simulink model "simple_streaming_txrx"  (Simulink 6.6)
settings: Solver=ode45  StartTime=0.0  StopTime=inf  RelTol=1e-3
InitFcn:
  | simple_streaming_init
StartFcn:
  | simple_streaming_init
undefined symbols (not defined in the file): dmf, gcbh, get, modConstellation_qam16, modConstellation_qam64, modConstellation_qpsk, rcosfir, symbolRomLen, txLSFR_initValues, txLSFR_polynomials, viqAvgLen, xlBlockLoadCallback, xlGetSimulinkPeriod
libraries: xbsIndex_r4 x506, commchan3 x2, commsink2 x1
(part 3 of 5)

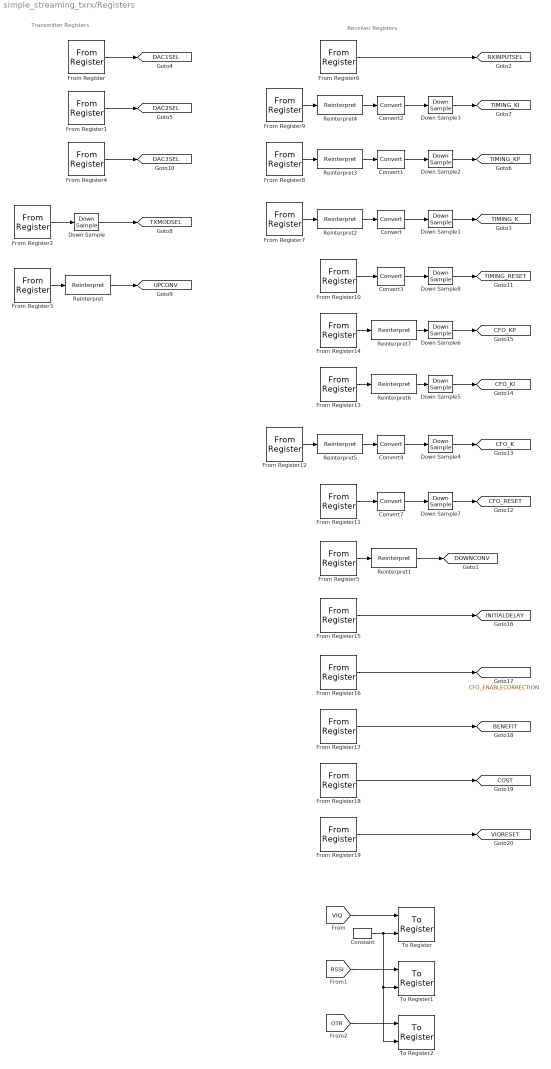
== system simple_streaming_txrx/Registers ==
  note: Transmitter Registers
  note: Receiver Registers
  Constant : xbsIndex_r4/Constant  arith_type=Boolean  const=1  n_bits=16  bin_pt=14  explicit_period=off  period=1  equ=P=C  opselect=C  inp2=PCIN>>17  opr=+  inp1=P  carry=CIN  dbl_ovrd=off  block_type=constant
      settings: block_version=10.1.2
  Convert : xbsIndex_r4/Convert  arith_type=Unsigned  n_bits=17  bin_pt=14  quantization=Truncate  overflow=Wrap  latency=0  dbl_ovrd=off  pipeline=off  block_type=convert
      settings: xl_area=[0 0 0 0 0 0 0]  block_version=10.1
  Convert1 : xbsIndex_r4/Convert  arith_type=Unsigned  n_bits=34  bin_pt=34  quantization=Truncate  overflow=Wrap  latency=0  dbl_ovrd=off  pipeline=off  block_type=convert
      settings: xl_area=[0 0 0 0 0 0 0]  block_version=10.1
  Convert2 : xbsIndex_r4/Convert  arith_type=Unsigned  n_bits=34  bin_pt=34  quantization=Truncate  overflow=Wrap  latency=0  dbl_ovrd=off  pipeline=off  block_type=convert
      settings: xl_area=[0 0 0 0 0 0 0]  block_version=10.1
  Convert3 : xbsIndex_r4/Convert  arith_type=Boolean  n_bits=17  bin_pt=14  quantization=Truncate  overflow=Wrap  latency=0  dbl_ovrd=off  pipeline=off  block_type=convert
      settings: xl_area=[0 0 0 0 0 0 0]  block_version=10.1
  Convert4 : xbsIndex_r4/Convert  arith_type=Unsigned  n_bits=17  bin_pt=10  quantization=Truncate  overflow=Wrap  latency=0  dbl_ovrd=off  pipeline=off  block_type=convert
      settings: xl_area=[0 0 0 0 0 0 0]  block_version=10.1
  Convert7 : xbsIndex_r4/Convert  arith_type=Boolean  n_bits=17  bin_pt=14  quantization=Truncate  overflow=Wrap  latency=0  dbl_ovrd=off  pipeline=off  block_type=convert
      settings: xl_area=[0 0 0 0 0 0 0]  block_version=10.1
  Down Sample{,1..8} (9 alike) : xbsIndex_r4/Down Sample  sample_ratio=8  sample_phase="Last Value of Frame  (most efficient)"  en=off  latency=1  dbl_ovrd=off  block_type=dsamp
      Down Sample settings: xl_area=[1 2 0 0 0 0 0]  block_version=10.1
      Down Sample1 settings: xl_area=[9 17 0 0 0 0 0]  block_version=10.1
      Down Sample2 settings: xl_area=[17 34 0 0 0 0 0]  block_version=10.1
      Down Sample3 settings: xl_area=[17 34 0 0 0 0 0]  block_version=10.1
      Down Sample4 settings: xl_area=[9 17 0 0 0 0 0]  block_version=10.1
      Down Sample5 settings: xl_area=[16 32 0 0 0 0 0]  block_version=10.1
      Down Sample6 settings: xl_area=[16 32 0 0 0 0 0]  block_version=10.1
      Down Sample7 settings: xl_area=[1 1 0 0 0 0 0]  block_version=10.1
      Down Sample8 settings: xl_area=[1 1 0 0 0 0 0]  block_version=10.1
  From Register : xbsIndex_r4/From Register  shared_memory_name='dac1Sel'  init=dac1Sel  period=1/8  ownership=Locally owned and initialized  arith_type=Unsigned  n_bits=2  bin_pt=0  dbl_ovrd=off  block_type=fromreg
      settings: AttributesFormatString=<< %<shared_memory_name> >>  infoedit="Register block that reads data to a shared memory register.  Delay of one sample period."  block_version=10.1
  From Register1 : xbsIndex_r4/From Register  shared_memory_name='dac2Sel'  init=dac2Sel  period=1/8  ownership=Locally owned and initialized  arith_type=Unsigned  n_bits=2  bin_pt=0  dbl_ovrd=off  block_type=fromreg
      settings: AttributesFormatString=<< %<shared_memory_name> >>  infoedit="Register block that reads data to a shared memory register.  Delay of one sample period."  block_version=10.1
  From Register10 : xbsIndex_r4/From Register  shared_memory_name='timingReset'  init=timingReset  period=1/8  ownership=Locally owned and initialized  arith_type=Unsigned  n_bits=1  bin_pt=0  dbl_ovrd=off  block_type=fromreg
      settings: AttributesFormatString=<< %<shared_memory_name> >>  infoedit="Register block that reads data to a shared memory register.  Delay of one sample period."  block_version=10.1
  From Register11 : xbsIndex_r4/From Register  shared_memory_name='cfoReset'  init=cfoReset  period=1/8  ownership=Locally owned and initialized  arith_type=Unsigned  n_bits=1  bin_pt=0  dbl_ovrd=off  block_type=fromreg
      settings: AttributesFormatString=<< %<shared_memory_name> >>  infoedit="Register block that reads data to a shared memory register.  Delay of one sample period."  block_version=10.1
  From Register12 : xbsIndex_r4/From Register  shared_memory_name='cfoK'  init=cfoK  period=1/8  ownership=Locally owned and initialized  arith_type=Unsigned  n_bits=32  bin_pt=0  dbl_ovrd=off  block_type=fromreg
      settings: AttributesFormatString=<< %<shared_memory_name> >>  infoedit="Register block that reads data to a shared memory register.  Delay of one sample period."  block_version=10.1
  From Register13 : xbsIndex_r4/From Register  shared_memory_name='cfoKI'  init=cfoKI  period=1/8  ownership=Locally owned and initialized  arith_type=Unsigned  n_bits=32  bin_pt=0  dbl_ovrd=off  block_type=fromreg
      settings: AttributesFormatString=<< %<shared_memory_name> >>  infoedit="Register block that reads data to a shared memory register.  Delay of one sample period."  block_version=10.1
  From Register14 : xbsIndex_r4/From Register  shared_memory_name='cfoKP'  init=cfoKP  period=1/8  ownership=Locally owned and initialized  arith_type=Unsigned  n_bits=32  bin_pt=0  dbl_ovrd=off  block_type=fromreg
      settings: AttributesFormatString=<< %<shared_memory_name> >>  infoedit="Register block that reads data to a shared memory register.  Delay of one sample period."  block_version=10.1
  From Register15 : xbsIndex_r4/From Register  shared_memory_name='initialDelay'  init=initialDelay  period=1/8  ownership=Locally owned and initialized  arith_type=Unsigned  n_bits=2  bin_pt=0  dbl_ovrd=off  block_type=fromreg
      settings: AttributesFormatString=<< %<shared_memory_name> >>  infoedit="Register block that reads data to a shared memory register.  Delay of one sample period."  block_version=10.1
  From Register16 : xbsIndex_r4/From Register  shared_memory_name='cfoEnable'  init=cfoEnable  period=1/8  ownership=Locally owned and initialized  arith_type=Unsigned  n_bits=1  bin_pt=0  dbl_ovrd=off  block_type=fromreg
      settings: AttributesFormatString=<< %<shared_memory_name> >>  infoedit="Register block that reads data to a shared memory register.  Delay of one sample period."  block_version=10.1
  From Register17 : xbsIndex_r4/From Register  shared_memory_name='otrBenefit'  init=benefit  period=1/8  ownership=Locally owned and initialized  arith_type=Unsigned  n_bits=32  bin_pt=0  dbl_ovrd=off  block_type=fromreg
      settings: AttributesFormatString=<< %<shared_memory_name> >>  infoedit="Register block that reads data to a shared memory register.  Delay of one sample period."  block_version=10.1
  From Register18 : xbsIndex_r4/From Register  shared_memory_name='otrCost'  init=cost  period=1/8  ownership=Locally owned and initialized  arith_type=Unsigned  n_bits=32  bin_pt=0  dbl_ovrd=off  block_type=fromreg
      settings: AttributesFormatString=<< %<shared_memory_name> >>  infoedit="Register block that reads data to a shared memory register.  Delay of one sample period."  block_version=10.1
  From Register19 : xbsIndex_r4/From Register  shared_memory_name='viqReset'  init=0  period=1/8  ownership=Locally owned and initialized  arith_type=Unsigned  n_bits=1  bin_pt=0  dbl_ovrd=off  block_type=fromreg
      settings: AttributesFormatString=<< %<shared_memory_name> >>  infoedit="Register block that reads data to a shared memory register.  Delay of one sample period."  block_version=10.1
  From Register2 : xbsIndex_r4/From Register  shared_memory_name='txModSel'  init=txModSel  period=1/8  ownership=Locally owned and initialized  arith_type=Unsigned  n_bits=2  bin_pt=0  dbl_ovrd=off  block_type=fromreg
      settings: AttributesFormatString=<< %<shared_memory_name> >>  infoedit="Register block that reads data to a shared memory register.  Delay of one sample period."  block_version=10.1
  From Register3 : xbsIndex_r4/From Register  shared_memory_name='upConv'  init=upConv  period=1/8  ownership=Locally owned and initialized  arith_type=Unsigned  n_bits=32  bin_pt=0  dbl_ovrd=off  block_type=fromreg
      settings: AttributesFormatString=<< %<shared_memory_name> >>  infoedit="Register block that reads data to a shared memory register.  Delay of one sample period."  block_version=10.1
  From Register4 : xbsIndex_r4/From Register  shared_memory_name='dac3Sel'  init=dac3Sel  period=1/8  ownership=Locally owned and initialized  arith_type=Unsigned  n_bits=1  bin_pt=0  dbl_ovrd=off  block_type=fromreg
      settings: AttributesFormatString=<< %<shared_memory_name> >>  infoedit="Register block that reads data to a shared memory register.  Delay of one sample period."  block_version=10.1
  From Register5 : xbsIndex_r4/From Register  shared_memory_name='downConv'  init=downConv  period=1/8  ownership=Locally owned and initialized  arith_type=Unsigned  n_bits=32  bin_pt=0  dbl_ovrd=off  block_type=fromreg
      settings: AttributesFormatString=<< %<shared_memory_name> >>  infoedit="Register block that reads data to a shared memory register.  Delay of one sample period."  block_version=10.1
  From Register6 : xbsIndex_r4/From Register  shared_memory_name='rxInputSel'  init=rxInputSel  period=1/8  ownership=Locally owned and initialized  arith_type=Unsigned  n_bits=2  bin_pt=0  dbl_ovrd=off  block_type=fromreg
      settings: AttributesFormatString=<< %<shared_memory_name> >>  infoedit="Register block that reads data to a shared memory register.  Delay of one sample period."  block_version=10.1
  From Register7 : xbsIndex_r4/From Register  shared_memory_name='timingK'  init=timingK  period=1/8  ownership=Locally owned and initialized  arith_type=Unsigned  n_bits=32  bin_pt=0  dbl_ovrd=off  block_type=fromreg
      settings: AttributesFormatString=<< %<shared_memory_name> >>  infoedit="Register block that reads data to a shared memory register.  Delay of one sample period."  block_version=10.1
  From Register8 : xbsIndex_r4/From Register  shared_memory_name='timingKP'  init=timingKP  period=1/8  ownership=Locally owned and initialized  arith_type=Unsigned  n_bits=32  bin_pt=0  dbl_ovrd=off  block_type=fromreg
      settings: AttributesFormatString=<< %<shared_memory_name> >>  infoedit="Register block that reads data to a shared memory register.  Delay of one sample period."  block_version=10.1
  From Register9 : xbsIndex_r4/From Register  shared_memory_name='timingKI'  init=timingKI  period=1/8  ownership=Locally owned and initialized  arith_type=Unsigned  n_bits=32  bin_pt=0  dbl_ovrd=off  block_type=fromreg
      settings: AttributesFormatString=<< %<shared_memory_name> >>  infoedit="Register block that reads data to a shared memory register.  Delay of one sample period."  block_version=10.1
  Reinterpret{,1,3..4,6..7} (6 alike) : xbsIndex_r4/Reinterpret  force_arith_type=on  arith_type=Unsigned  force_bin_pt=on  bin_pt=32  block_type=reinterpret
      settings: infoedit="Changes signal type without altering the binary representation.   You can changed the signal between signed and unsigned, and relocate the binary point.<P><P>Hardware notes: In hardware this block costs nothing.<P><P>Example:  Suppose the input is 6 bits wide, signed, with 2 fractional bits, and the output is forced to unsigned with 0 fractional bits.  Then an input of -2.0 (1110.00 in binary 2's complement) becomes an output of 56 (111000 in binary)."  block_version=10.1
  Reinterpret2 : xbsIndex_r4/Reinterpret  force_arith_type=on  arith_type=Unsigned  force_bin_pt=on  bin_pt=29  block_type=reinterpret
      settings: infoedit="Changes signal type without altering the binary representation.   You can changed the signal between signed and unsigned, and relocate the binary point.<P><P>Hardware notes: In hardware this block costs nothing.<P><P>Example:  Suppose the input is 6 bits wide, signed, with 2 fractional bits, and the output is forced to unsigned with 0 fractional bits.  Then an input of -2.0 (1110.00 in binary 2's complement) becomes an output of 56 (111000 in binary)."  block_version=10.1
  Reinterpret5 : xbsIndex_r4/Reinterpret  force_arith_type=on  arith_type=Unsigned  force_bin_pt=on  bin_pt=25  block_type=reinterpret
      settings: infoedit="Changes signal type without altering the binary representation.   You can changed the signal between signed and unsigned, and relocate the binary point.<P><P>Hardware notes: In hardware this block costs nothing.<P><P>Example:  Suppose the input is 6 bits wide, signed, with 2 fractional bits, and the output is forced to unsigned with 0 fractional bits.  Then an input of -2.0 (1110.00 in binary 2's complement) becomes an output of 56 (111000 in binary)."  block_version=10.1
  To Register : xbsIndex_r4/To Register  shared_memory_name='viq'  init=0  ownership=Locally owned and initialized  explicit_data_type=on  arith_type=Unsigned  n_bits=32  bin_pt=0  dbl_ovrd=off  block_type=toreg
      settings: AttributesFormatString=<< %<shared_memory_name> >>  infoedit="Register block that writes data to a shared memory register.  Delay of one sample period."  block_version=10.1.2
  To Register1 : xbsIndex_r4/To Register  shared_memory_name='rssi'  init=0  ownership=Locally owned and initialized  explicit_data_type=on  arith_type=Unsigned  n_bits=32  bin_pt=0  dbl_ovrd=off  block_type=toreg
      settings: AttributesFormatString=<< %<shared_memory_name> >>  infoedit="Register block that writes data to a shared memory register.  Delay of one sample period."  block_version=10.1.2
  To Register2 : xbsIndex_r4/To Register  shared_memory_name='otr'  init=0  ownership=Locally owned and initialized  explicit_data_type=on  arith_type=Unsigned  n_bits=32  bin_pt=0  dbl_ovrd=off  block_type=toreg
      settings: AttributesFormatString=<< %<shared_memory_name> >>  infoedit="Register block that writes data to a shared memory register.  Delay of one sample period."  block_version=10.1.2
  tag scope: BENEFIT=global, CFO_ENABLECORRECTION=global, CFO_K=global, CFO_KI=global, CFO_KP=global, CFO_RESET=global, COST=global, DAC1SEL=global, DAC2SEL=global, DAC3SEL=global, DOWNCONV=global, INITIALDELAY=global, RXINPUTSEL=global, TIMING_K=global, TIMING_KI=global, TIMING_KP=global, TIMING_RESET=global, TXMODSEL=global, UPCONV=global, VIQRESET=global
  wires:
  From Register/1 -> [DAC1SEL]
  From Register1/1 -> [DAC2SEL]
  From Register2/1 -> Down Sample/1
  Down Sample/1 -> [TXMODSEL]
  From Register3/1 -> Reinterpret/1
  Reinterpret/1 -> [UPCONV]
  From Register4/1 -> [DAC3SEL]
  From Register5/1 -> Reinterpret1/1
  Reinterpret1/1 -> [DOWNCONV]
  From Register6/1 -> [RXINPUTSEL]
  From Register7/1 -> Reinterpret2/1
  Reinterpret2/1 -> Convert/1
  Convert/1 -> Down Sample1/1
  From Register8/1 -> Reinterpret3/1
  Reinterpret3/1 -> Convert1/1
  Convert1/1 -> Down Sample2/1
  From Register9/1 -> Reinterpret4/1
  Reinterpret4/1 -> Convert2/1
  Convert2/1 -> Down Sample3/1
  From Register10/1 -> Convert3/1
  Convert3/1 -> Down Sample8/1
  Down Sample1/1 -> [TIMING_K]
  Down Sample2/1 -> [TIMING_KP]
  Down Sample3/1 -> [TIMING_KI]
  From Register12/1 -> Reinterpret5/1
  Reinterpret5/1 -> Convert4/1
  Convert4/1 -> Down Sample4/1
  From Register13/1 -> Reinterpret6/1
  Reinterpret6/1 -> Down Sample5/1
  From Register14/1 -> Reinterpret7/1
  Reinterpret7/1 -> Down Sample6/1
  From Register11/1 -> Convert7/1
  Convert7/1 -> Down Sample7/1
  Down Sample4/1 -> [CFO_K]
  Down Sample5/1 -> [CFO_KI]
  Down Sample6/1 -> [CFO_KP]
  Down Sample7/1 -> [CFO_RESET]
  Down Sample8/1 -> [TIMING_RESET]
  From Register15/1 -> [INITIALDELAY]
  From Register16/1 -> [CFO_ENABLECORRECTION]
  From Register17/1 -> [BENEFIT]
  From Register18/1 -> [COST]
  [VIQ] -> To Register/1
  [RSSI] -> To Register1/1
  [OTR] -> To Register2/1
  Constant/1 -> To Register1/2, To Register2/2, To Register/2
  From Register19/1 -> [VIQRESET]

== system simple_streaming_txrx/Transmitter ==
  Interpolate : Subsystem
  Random Symbols : Subsystem
  Register : xbsIndex_r4/Register  init=0  rst=off  en=off  dbl_ovrd=off  block_type=register
      settings: xl_area=[8 16 0 0 0 0 0]  block_version=10.1
  Register1 : xbsIndex_r4/Register  init=0  rst=off  en=off  dbl_ovrd=off  block_type=register
      settings: xl_area=[8 16 0 0 0 0 0]  block_version=10.1
  TX_I : xbsIndex_r4/Gateway Out  hdl_port=on  timing_constraint=None  locs_specified=off  LOCs={}  block_type=gatewayout
      settings: infoedit="Gateway out block.  Converts Xilinx fixed point inputs into ouputs of type Simulink integer, double, or fixed point.<P><P>Hardware notes:  In hardware these blocks become top level output ports or are discarded, depending on how they are configured."  xl_area=[0 0 0 0 16 0 0]  block_version=10.1
  TX_Q : xbsIndex_r4/Gateway Out  hdl_port=on  timing_constraint=None  locs_specified=off  LOCs={}  block_type=gatewayout
      settings: infoedit="Gateway out block.  Converts Xilinx fixed point inputs into ouputs of type Simulink integer, double, or fixed point.<P><P>Hardware notes:  In hardware these blocks become top level output ports or are discarded, depending on how they are configured."  xl_area=[0 0 0 0 16 0 0]  block_version=10.1
  Upconverter : Subsystem
  Upconverted : Outport
  IF I : Outport  Port=2
  IF Q : Outport  Port=3
  tag scope: Symbols_Filt_I=global, Symbols_Filt_Q=global, Symbols_Tx_I=global, Symbols_Tx_Q=global, Upconverted=global
  wires:
  Random Symbols/1(I) -> [Symbols_Tx_I], Interpolate/1(I)
  Random Symbols/2(Q) -> [Symbols_Tx_Q], Interpolate/2(Q)
  Interpolate/1(" I") -> [Symbols_Filt_I], Upconverter/1(I)
  Interpolate/2(" Q") -> [Symbols_Filt_Q], Upconverter/2(Q)
  Upconverter/1(" Mixed") -> [Upconverted], Upconverted/1
  Upconverter/2(" I") -> Register/1
  Upconverter/3(" Q") -> Register1/1
  TX_I/1 -> IF I/1
  TX_Q/1 -> IF Q/1
  Register/1 -> TX_I/1
  Register1/1 -> TX_Q/1

== system simple_streaming_txrx/Receiver/AGC Hook ==
  I : Inport
  Q : Inport  Port=2
  Coarse : Subsystem
  Fine : Subsystem
  IO : Outport
  OO : Outport  Port=2
  wires:
  I/1 -> IO/1, Fine/1(I)
  Q/1 -> OO/1, Fine/2(Q)

== system simple_streaming_txrx/Receiver/Carrier Recovery ==
  I : Inport
  Q : Inport  Port=2
  2nd Order Filter : Subsystem
  Convert : xbsIndex_r4/Convert  arith_type=Boolean  n_bits=16  bin_pt=14  quantization=Truncate  overflow=Wrap  latency=0  dbl_ovrd=off  pipeline=off  block_type=convert
      settings: xl_area=[0 0 0 0 0 0 0]  block_version=10.1
  Inverter : xbsIndex_r4/Inverter  en=off  latency=0  dbl_ovrd=off  block_type=inv
      settings: xl_area=[0 0 0 0 0 0 0]  block_version=10.1
  Mult2 : xbsIndex_r4/Mult  precision=User Defined  arith_type="Signed  (2's comp)"  n_bits=32  bin_pt=31  quantization=Truncate  overflow=Flag as error  en=off  latency=3  dbl_ovrd=off  use_behavioral_HDL=off  use_embedded=on  opt=Speed  optimum_pipeline=off  pipeline=on  use_rpm=on  placement_style=Rectangular shape  block_type=mult
      settings: infoedit=Hardware notes: To use the internal pipeline stage of the dedicated multiplier you must select 'Pipeline for maximum performance'.  xl_area=[59 104 0 100 0 3 0]  block_version=10.1
  Phase Error Detector : Subsystem
  Register : xbsIndex_r4/Register  init=0  rst=on  en=off  dbl_ovrd=off  block_type=register
      settings: xl_area=[16 32 0 0 0 0 0]  block_version=10.1
  Up Sample : xbsIndex_r4/Up Sample  sample_ratio=8  copy_samples=on  dbl_ovrd=off  block_type=usamp
      settings: infoedit="Up samples input data.  Inserted values  can be zeros or copies of the most recent input sample.<P><P>Hardware notes: No hardware is needed if inserted values are copies of the input sample; otherwise, a mux and single bit flip-flop are used."  xl_area=[0 0 0 0 0 0 0]  block_version=10.1
  " phase inc" : Outport
  tag scope: CFOINC=global, PHASEERROR=global
  wires:
  Phase Error Detector/1(Err) -> 2nd Order Filter/1(Phase Error), [PHASEERROR]
  [CFO_RESET] -> 2nd Order Filter/2(Reset)
  Up Sample/1 -> Register/1
  2nd Order Filter/1(Phase Inc) -> Mult2/1
  I/1 -> Phase Error Detector/1(I)
  Q/1 -> Phase Error Detector/2(Q)
  [CFO_K] -> Mult2/2
  Mult2/1 -> Up Sample/1, [CFOINC]
  Register/1 -> " phase inc"/1
  [CFO_ENABLECORRECTION] -> Inverter/1
  Inverter/1 -> Convert/1
  Convert/1 -> Register/2

== system simple_streaming_txrx/Receiver/Decimate & Filter ==
  I : Inport
  Q : Inport  Port=2
  Convert1 : xbsIndex_r4/Convert  arith_type="Signed  (2's comp)"  n_bits=16  bin_pt=15  quantization=Truncate  overflow=Wrap  latency=0  dbl_ovrd=off  pipeline=off  block_type=convert
      settings: xl_area=[0 0 0 0 0 0 0]  block_version=10.1
  Convert2 : xbsIndex_r4/Convert  arith_type="Signed  (2's comp)"  n_bits=16  bin_pt=15  quantization=Truncate  overflow=Wrap  latency=0  dbl_ovrd=off  pipeline=off  block_type=convert
      settings: xl_area=[0 0 0 0 0 0 0]  block_version=10.1
  Convert3 : xbsIndex_r4/Convert  arith_type="Signed  (2's comp)"  n_bits=16  bin_pt=15  quantization=Truncate  overflow=Wrap  latency=0  dbl_ovrd=off  pipeline=off  block_type=convert
      settings: xl_area=[0 0 0 0 0 0 0]  block_version=10.1
  I MF1 : Subsystem  mask{h_in=rcosfir(.3, 4, 8, 1,'sqrt'), polyphaseBranches=8, data_samplePeriod=1/8, coeff_prec=14, coeff_bp=13, multLatency=1, mult_prec=18, mult_bp=17, add_prec=16, add_bp=14}
      mask prompts: h_in "Filter Coefficients"; polyphaseBranches "Interpolation Rate"; data_samplePeriod "Input Sample Period"; coeff_prec "Coefficients - Num Bits"; coeff_bp "Coefficients - Binary Point"; multLatency "Multiplier Latency"; mult_prec "Multiplier - Num Bits"; mult_bp "Multiplier - Binary Point"; add_prec "Final Adder - Num Bits"; add_bp "Final Adder - Binary Point"
      mask help:
      | This block implements a decimating polyphase FIR filter. In this version,
      | the decimation rate must be 8, and the filter must be of length 64.
      mask init:
      | h = reshape(reshape(h_in(1:64),8,8)',1,64);
      | subFilterLength = 8;
  I MF2 : Subsystem  mask{h_in=rcosfir(.3, 4, 8, 1,'sqrt'), polyphaseBranches=8, data_samplePeriod=1/8, coeff_prec=14, coeff_bp=13, multLatency=1, mult_prec=18, mult_bp=17, add_prec=16, add_bp=14}
      mask prompts: h_in "Filter Coefficients"; polyphaseBranches "Interpolation Rate"; data_samplePeriod "Input Sample Period"; coeff_prec "Coefficients - Num Bits"; coeff_bp "Coefficients - Binary Point"; multLatency "Multiplier Latency"; mult_prec "Multiplier - Num Bits"; mult_bp "Multiplier - Binary Point"; add_prec "Final Adder - Num Bits"; add_bp "Final Adder - Binary Point"
      mask help:
      | This block implements a decimating polyphase FIR filter. In this version,
      | the decimation rate must be 8, and the filter must be of length 64.
      mask init:
      | h = reshape(reshape(h_in(1:64),8,8)',1,64);
      | subFilterLength = 8;
  Scale : xbsIndex_r4/Scale  scale_factor=1  dbl_ovrd=off  block_type=scale
      settings: infoedit=Scales input by a power of two by adjusting the binary point position.<P><P>Hardware notes: In hardware this block costs nothing.  block_version=10.1
  Scale1 : xbsIndex_r4/Scale  scale_factor=0  dbl_ovrd=off  block_type=scale
      settings: infoedit=Scales input by a power of two by adjusting the binary point position.<P><P>Hardware notes: In hardware this block costs nothing.  block_version=10.1
  Scale2 : xbsIndex_r4/Scale  scale_factor=1  dbl_ovrd=off  block_type=scale
      settings: infoedit=Scales input by a power of two by adjusting the binary point position.<P><P>Hardware notes: In hardware this block costs nothing.  block_version=10.1
  Scope : Scope  NumInputPorts=6
      settings: YMin=-0.75~-0.75~-1~-1.5~-1.5~-1  YMax=0.75~0.75~0.75~1.5~1.5~0.75  SaveName=ScopeData4
  dMF : Subsystem  mask{h_in=dmf*2, polyphaseBranches=8, data_samplePeriod=1/8, coeff_prec=14, coeff_bp=13, multLatency=1, mult_prec=18, mult_bp=17, add_prec=16, add_bp=14}
      mask prompts: h_in "Filter Coefficients"; polyphaseBranches "Interpolation Rate"; data_samplePeriod "Input Sample Period"; coeff_prec "Coefficients - Num Bits"; coeff_bp "Coefficients - Binary Point"; multLatency "Multiplier Latency"; mult_prec "Multiplier - Num Bits"; mult_bp "Multiplier - Binary Point"; add_prec "Final Adder - Num Bits"; add_bp "Final Adder - Binary Point"
      mask help:
      | This block implements a decimating polyphase FIR filter. In this version,
      | the decimation rate must be 8, and the filter must be of length 64.
      mask init:
      | h = reshape(reshape(h_in(1:64),8,8)',1,64);
      | subFilterLength = 8;
  " I" : Outport
  " Q" : Outport  Port=2
  " dI" : Outport  Port=3
  wires:
  I/1 -> I MF1/1(X), dMF/1(X)
  I MF1/1(Y) -> Scale/1, Scope/1
  Q/1 -> I MF2/1(X)
  Scale/1 -> Convert3/1, Scope/4
  Scale2/1 -> Convert1/1, Scope/5
  Convert3/1 -> " I"/1
  Convert1/1 -> " Q"/1
  I MF2/1(Y) -> Scale2/1, Scope/2
  dMF/1(Y) -> Scale1/1, Scope/3
  Scale1/1 -> Convert2/1, Scope/6
  Convert2/1 -> " dI"/1

== system simple_streaming_txrx/Receiver/Downconverter ==
  Mixed : Inport
  SEL : Inport  Port=2
  I : Inport  Port=3
  Q : Inport  Port=4
  Phase Inc : Inport  Port=5
  AddSub : xbsIndex_r4/AddSub  mode=Addition  use_carryin=off  use_carryout=off  en=off  latency=0  precision=User Defined  arith_type=Unsigned  n_bits=32  bin_pt=32  quantization=Truncate  overflow=Wrap  dbl_ovrd=off  use_behavioral_HDL=on  pipelined=off  use_rpm=on  block_type=addsub
      settings: xl_area=[16 0 0 31 0 0 0]  block_version=10.1
  ComplexMult : Subsystem
  Inverter1 : xbsIndex_r4/Inverter  en=off  latency=0  dbl_ovrd=off  block_type=inv
      settings: xl_area=[0 0 0 0 0 0 0]  block_version=10.1
  Mux1 : xbsIndex_r4/Mux  inputs=3  en=off  latency=1  precision=Full  arith_type="Signed  (2's comp)"  n_bits=8  bin_pt=2  quantization=Truncate  overflow=Wrap  dbl_ovrd=off  block_type=mux
      settings: xl_area=[18 18 0 36 0 0 0]  block_version=10.1
  Mux2 : xbsIndex_r4/Mux  inputs=3  en=off  latency=1  precision=Full  arith_type="Signed  (2's comp)"  n_bits=8  bin_pt=2  quantization=Truncate  overflow=Wrap  dbl_ovrd=off  block_type=mux
      settings: xl_area=[18 18 0 36 0 0 0]  block_version=10.1
  i1i1 : xbsIndex_r4/Mult  precision=User Defined  arith_type="Signed  (2's comp)"  n_bits=18  bin_pt=17  quantization=Truncate  overflow=Flag as error  en=off  latency=1  dbl_ovrd=off  use_behavioral_HDL=off  use_embedded=on  opt=Speed  optimum_pipeline=off  pipeline=on  use_rpm=on  placement_style=Rectangular shape  block_type=mult
      settings: infoedit=Hardware notes: To use the internal pipeline stage of the dedicated multiplier you must select 'Pipeline for maximum performance'.  xl_area=[9 -11 0 18 0 1 0]  block_version=10.1
  i1i2 : xbsIndex_r4/Mult  precision=User Defined  arith_type="Signed  (2's comp)"  n_bits=18  bin_pt=17  quantization=Truncate  overflow=Flag as error  en=off  latency=1  dbl_ovrd=off  use_behavioral_HDL=off  use_embedded=on  opt=Speed  optimum_pipeline=off  pipeline=on  use_rpm=on  placement_style=Rectangular shape  block_type=mult
      settings: infoedit=Hardware notes: To use the internal pipeline stage of the dedicated multiplier you must select 'Pipeline for maximum performance'.  xl_area=[9 -11 0 18 0 1 0]  block_version=10.1
  myDDS : Subsystem
  " I" : Outport
  " Q" : Outport  Port=2
  tag scope: dCarrier_I=global
  wires:
  Mixed/1 -> i1i2/1, i1i1/1
  AddSub/1 -> myDDS/1(phase inc)
  Phase Inc/1 -> AddSub/2
  [DOWNCONV] -> AddSub/1
  myDDS/1(sin) -> Inverter1/1
  myDDS/2(cos) -> i1i2/2, [dCarrier_I], ComplexMult/1(A I)
  Mux1/1 -> " I"/1
  Mux2/1 -> " Q"/1
  SEL/1 -> Mux1/1, Mux2/1
  i1i2/1 -> Mux1/3, Mux1/2
  i1i1/1 -> Mux2/3, Mux2/2
  I/1 -> ComplexMult/3(B I)
  Q/1 -> ComplexMult/4(B Q)
  ComplexMult/1(I) -> Mux1/4
  ComplexMult/2(Q) -> Mux2/4
  Inverter1/1 -> i1i1/2, ComplexMult/2(A Q)

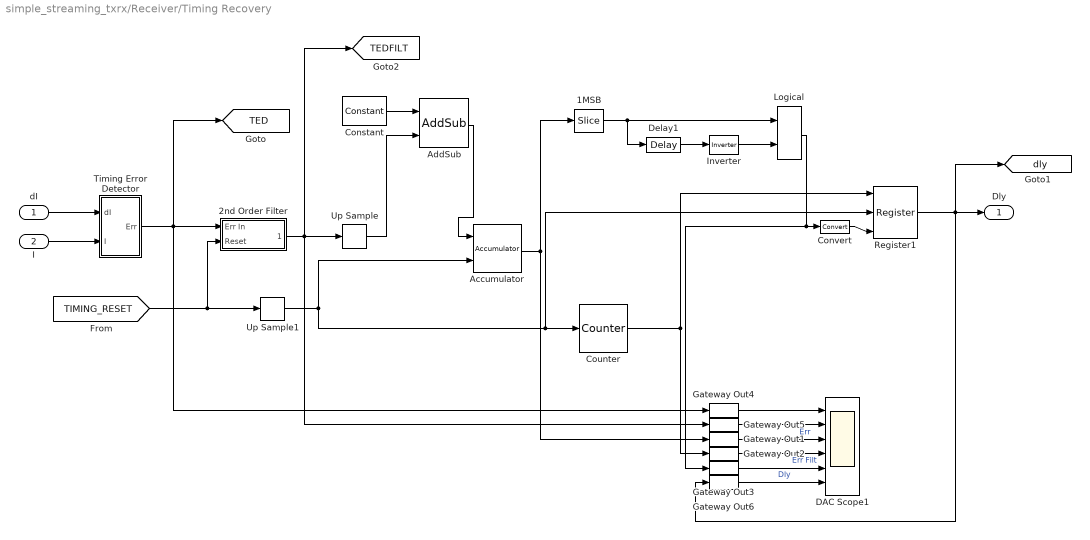
== system simple_streaming_txrx/Receiver/Timing Recovery ==
  dI : Inport
  I : Inport  Port=2
  1MSB : xbsIndex_r4/Slice  nbits=1  boolean_output=off  mode=Upper Bit Location + Width  bit1=0  base1=MSB of Input  bit0=0  base0=LSB of Input  dbl_ovrd=off  block_type=slice
      settings: infoedit="Extracts a given range of bits from each input sample and presents it at the output.  The output type is ordinarily unsigned with binary point at zero, but can be Boolean when the slice is one bit wide.<P><P>Hardware notes: In hardware this block costs nothing."  block_version=10.1
  2nd Order Filter : Subsystem
  Accumulator : xbsIndex_r4/Accumulator  operation=Add  n_bits=32  overflow=Wrap  scale=1  rst=on  hasbypass=off  en=off  dbl_ovrd=off  use_behavioral_HDL=on  block_type=accum
      settings: infoedit="Adder or subtractor-based accumulator.   Output type and binary point position match the input.<P><P>Hardware notes: When \"Reinitialize with input 'b' on reset\" is selected, the accumulator is forced to run at the system rate even if the input 'b' is running at a slower rate."  xl_area=[16 32 0 32 0 0 0]  block_version=10.1
  AddSub : xbsIndex_r4/AddSub  mode=Subtraction  use_carryin=off  use_carryout=off  en=off  latency=0  precision=User Defined  arith_type="Signed  (2's comp)"  n_bits=32  bin_pt=31  quantization=Truncate  overflow=Wrap  dbl_ovrd=off  use_behavioral_HDL=on  pipelined=off  use_rpm=on  block_type=addsub
      settings: xl_area=[2 0 0 4 0 0 0]  block_version=10.1
  Constant : xbsIndex_r4/Constant  arith_type=Unsigned  const=1/4  n_bits=4  bin_pt=3  explicit_period=on  period=1/8  equ=P=C  opselect=C  inp2=PCIN>>17  opr=+  inp1=P  carry=CIN  dbl_ovrd=off  block_type=constant
      settings: block_version=10.1
  Convert : xbsIndex_r4/Convert  arith_type=Boolean  n_bits=8  bin_pt=6  quantization=Truncate  overflow=Wrap  latency=0  dbl_ovrd=off  pipeline=off  block_type=convert
      settings: xl_area=[0 0 0 0 0 0 0]  block_version=10.1
  Counter : xbsIndex_r4/Counter  cnt_type=Free Running  cnt_to=Inf  operation=Up  start_count=0  cnt_by_val=1  arith_type=Unsigned  n_bits=3  bin_pt=0  load_pin=off  rst=on  en=off  explicit_period=off  period=1/8  dbl_ovrd=off  use_behavioral_HDL=off  use_rpm=on  block_type=counter
      settings: xl_area=[3 3 0 3 0 0 0]  block_version=10.1
  DAC Scope1 : Scope  NumInputPorts=6
      settings: YMin=-0.4~-0.0075~-1~0~0~-1  YMax=0.4~0.0075~1~7~1~1  SaveName=ScopeData3
  Delay1 : xbsIndex_r4/Delay  en=off  latency=1  dbl_ovrd=off  reg_retiming=off  block_type=delay
      settings: xl_area=[1 1 0 0 0 0 0]  block_version=10.1
  Gateway Out{1..6} (6 alike) : xbsIndex_r4/Gateway Out  hdl_port=off  timing_constraint=None  locs_specified=off  LOCs={}  block_type=gatewayout
      settings: infoedit="Gateway out block.  Converts Xilinx fixed point inputs into ouputs of type Simulink integer, double, or fixed point.<P><P>Hardware notes:  In hardware these blocks become top level output ports or are discarded, depending on how they are configured."  xl_area=[0 0 0 0 0 0 0]  block_version=10.1
  Inverter : xbsIndex_r4/Inverter  en=off  latency=0  dbl_ovrd=off  block_type=inv
      settings: xl_area=[0 0 0 0 0 0 0]  block_version=10.1
  Logical : xbsIndex_r4/Logical  logical_function=AND  inputs=2  en=off  latency=0  precision=Full  arith_type=Unsigned  n_bits=8  bin_pt=2  align_bp=on  dbl_ovrd=off  block_type=logical
      settings: xl_area=[1 0 0 1 0 0 0]  block_version=10.1
  Register1 : xbsIndex_r4/Register  init=0  rst=on  en=on  dbl_ovrd=off  block_type=register
      settings: xl_area=[2 3 0 0 0 0 0]  block_version=10.1
  Timing Error Detector : Subsystem
  Up Sample : xbsIndex_r4/Up Sample  sample_ratio=8  copy_samples=on  dbl_ovrd=off  block_type=usamp
      settings: infoedit="Up samples input data.  Inserted values  can be zeros or copies of the most recent input sample.<P><P>Hardware notes: No hardware is needed if inserted values are copies of the input sample; otherwise, a mux and single bit flip-flop are used."  xl_area=[0 0 0 0 0 0 0]  block_version=10.1
  Up Sample1 : xbsIndex_r4/Up Sample  sample_ratio=8  copy_samples=on  dbl_ovrd=off  block_type=usamp
      settings: infoedit="Up samples input data.  Inserted values  can be zeros or copies of the most recent input sample.<P><P>Hardware notes: No hardware is needed if inserted values are copies of the input sample; otherwise, a mux and single bit flip-flop are used."  xl_area=[0 0 0 0 0 0 0]  block_version=10.1
  Dly : Outport
  tag scope: TED=global, TEDFILT=global, dly=global
  wires:
  Timing Error Detector/1(Err) -> 2nd Order Filter/1(Err In), Gateway Out4/1, [TED]
  [TIMING_RESET] -> 2nd Order Filter/2(Reset), Up Sample1/1
  I/1 -> Timing Error Detector/2(I)
  dI/1 -> Timing Error Detector/1(dI)
  2nd Order Filter/1(Err Filt) -> Up Sample/1, Gateway Out5/1, [TEDFILT]
  Delay1/1 -> Inverter/1
  1MSB/1 -> Logical/1, Delay1/1
  Inverter/1 -> Logical/2
  Accumulator/1 -> Gateway Out1/1, 1MSB/1
  Counter/1 -> Register1/1, Gateway Out2/1
  Logical/1 -> Convert/1, Gateway Out3/1
  Register1/1 -> Dly/1, [dly], Gateway Out6/1
  Convert/1 -> Register1/3
  Gateway Out4/1 -> DAC Scope1/1
  Gateway Out5/1 -> DAC Scope1/2
  Gateway Out1/1 -> DAC Scope1/3  "Err"
  Gateway Out2/1 -> DAC Scope1/4  "Err Filt"
  Gateway Out3/1 -> DAC Scope1/5  "Dly"
  Constant/1 -> AddSub/1
  Up Sample/1 -> AddSub/2
  AddSub/1 -> Accumulator/1
  Gateway Out6/1 -> DAC Scope1/6
  Up Sample1/1 -> Accumulator/2, Counter/1, Register1/2

== system simple_streaming_txrx/Receiver/Variable Delay ==
  D : Inport
  dly : Inport  Port=2
  ASR : xbsIndex_r4/Addressable Shift Register  infer_latency=on  depth=2  initVector=[0]  en=off  dbl_ovrd=off  use_behavioral_HDL=off  use_rpm=on  block_type=addrsr
      settings: infoedit="Delay of configurable length.  Any element in the delay line can be addressed and driven onto the output port.<br><br>Hardware notes: Implemented using SRL16s.  If Virtex-4, Virtex-II or Spartan-3 devices are used, multiple SRLC16s are cascaded together."  xl_area=[7 0 0 14 0 0 0]  block_version=10.1
  Q : Outport
  wires:
  D/1 -> ASR/1
  ASR/1 -> Q/1
  dly/1 -> ASR/2

== system simple_streaming_txrx/Receiver/Variable Delay1 ==
  D : Inport
  dly : Inport  Port=2
  ASR : xbsIndex_r4/Addressable Shift Register  infer_latency=on  depth=2  initVector=[0]  en=off  dbl_ovrd=off  use_behavioral_HDL=off  use_rpm=on  block_type=addrsr
      settings: infoedit="Delay of configurable length.  Any element in the delay line can be addressed and driven onto the output port.<br><br>Hardware notes: Implemented using SRL16s.  If Virtex-4, Virtex-II or Spartan-3 devices are used, multiple SRLC16s are cascaded together."  xl_area=[7 0 0 14 0 0 0]  block_version=10.1
  Q : Outport
  wires:
  dly/1 -> ASR/2
  ASR/1 -> Q/1
  D/1 -> ASR/1

== system simple_streaming_txrx/Receiver/Variable Delay2 ==
  D : Inport
  dly : Inport  Port=2
  ASR : xbsIndex_r4/Addressable Shift Register  infer_latency=on  depth=2  initVector=[0]  en=off  dbl_ovrd=off  use_behavioral_HDL=off  use_rpm=on  block_type=addrsr
      settings: infoedit="Delay of configurable length.  Any element in the delay line can be addressed and driven onto the output port.<br><br>Hardware notes: Implemented using SRL16s.  If Virtex-4, Virtex-II or Spartan-3 devices are used, multiple SRLC16s are cascaded together."  xl_area=[7 0 0 14 0 0 0]  block_version=10.1
  Q : Outport
  wires:
  D/1 -> ASR/1
  ASR/1 -> Q/1
  dly/1 -> ASR/2

== system simple_streaming_txrx/Transmitter/Interpolate ==
  I : Inport
  Q : Inport  Port=2
  Polyphase Interpolator2 : Subsystem  mask{h=rcosfir(.3, 4, 8, 1,'sqrt'), polyphaseBranches=8, data_samplePeriod=1, coeff_prec=14, coeff_bp=13, multLatency=1, mult_prec=18, mult_bp=17, add_prec=16, add_bp=15}
      mask prompts: h "Filter Coefficients"; polyphaseBranches "Interpolation Rate"; data_samplePeriod "Input Sample Period"; coeff_prec "Coefficients - Num Bits"; coeff_bp "Coefficients - Binary Point"; multLatency "Multiplier Latency"; mult_prec "Multiplier - Num Bits"; mult_bp "Multiplier - Binary Point"; add_prec "Final Adder - Num Bits"; add_bp "Final Adder - Binary Point"
      mask help:
      | This block implements a interpolating polyphase FIR filter. In this version,
      | the interpolation rate must be 8, and the filter must be of length 64.
      mask init:
      | subFilterLength = 8;
  Polyphase Interpolator3 : Subsystem  mask{h=rcosfir(.3, 4, 8, 1,'sqrt'), polyphaseBranches=8, data_samplePeriod=1, coeff_prec=14, coeff_bp=13, multLatency=1, mult_prec=18, mult_bp=17, add_prec=16, add_bp=15}
      mask prompts: h "Filter Coefficients"; polyphaseBranches "Interpolation Rate"; data_samplePeriod "Input Sample Period"; coeff_prec "Coefficients - Num Bits"; coeff_bp "Coefficients - Binary Point"; multLatency "Multiplier Latency"; mult_prec "Multiplier - Num Bits"; mult_bp "Multiplier - Binary Point"; add_prec "Final Adder - Num Bits"; add_bp "Final Adder - Binary Point"
      mask help:
      | This block implements a interpolating polyphase FIR filter. In this version,
      | the interpolation rate must be 8, and the filter must be of length 64.
      mask init:
      | subFilterLength = 8;
  " I" : Outport
  " Q" : Outport  Port=2
  wires:
  I/1 -> Polyphase Interpolator2/1(X)
  Q/1 -> Polyphase Interpolator3/1(X)
  Polyphase Interpolator2/1(Y) -> " I"/1
  Polyphase Interpolator3/1(Y) -> " Q"/1

== system simple_streaming_txrx/Transmitter/Random Symbols ==
  6bit Datasource : Subsystem
  Convert : xbsIndex_r4/Convert  arith_type="Signed  (2's comp)"  n_bits=16  bin_pt=15  quantization=Truncate  overflow=Wrap  latency=0  dbl_ovrd=off  pipeline=off  block_type=convert
      settings: xl_area=[0 0 0 0 0 0 0]  block_version=10.1
  Convert1 : xbsIndex_r4/Convert  arith_type="Signed  (2's comp)"  n_bits=16  bin_pt=15  quantization=Truncate  overflow=Wrap  latency=0  dbl_ovrd=off  pipeline=off  block_type=convert
      settings: xl_area=[0 0 0 0 0 0 0]  block_version=10.1
  Modulation : Subsystem
  I : Outport
  Q : Outport  Port=2
  wires:
  6bit Datasource/1(I) -> Modulation/2(I Bits)
  6bit Datasource/2(Q) -> Modulation/3(Q Bits)
  Modulation/1(I) -> Convert/1
  Modulation/2(Q) -> Convert1/1
  Convert/1 -> I/1
  Convert1/1 -> Q/1
  [TXMODSEL] -> Modulation/1(Mod Sel)

== system simple_streaming_txrx/Transmitter/Upconverter ==
  I : Inport
  Q : Inport  Port=2
  ComplexMult : Subsystem
  Re[A*B] : Subsystem
  myDDS : Subsystem
  " Mixed" : Outport
  " I" : Outport  Port=2
  " Q" : Outport  Port=3
  tag scope: Carrier_I=global
  wires:
  I/1 -> Re[A*B]/1(A I), ComplexMult/1(A I)
  Q/1 -> Re[A*B]/2(A Q), ComplexMult/2(A Q)
  myDDS/2(cos) -> [Carrier_I], Re[A*B]/3(B I), ComplexMult/3(B I)
  myDDS/1(sin) -> Re[A*B]/4(B Q), ComplexMult/4(B Q)
  [UPCONV] -> myDDS/1(phase inc)
  Re[A*B]/1(Out) -> " Mixed"/1
  ComplexMult/1(I) -> " I"/1
  ComplexMult/2(Q) -> " Q"/1

== system simple_streaming_txrx/Receiver/AGC Hook/Coarse ==
  Accumulator : xbsIndex_r4/Accumulator  operation=Add  n_bits=32  overflow=Saturate  scale=1  rst=off  hasbypass=off  en=off  dbl_ovrd=off  use_behavioral_HDL=on  block_type=accum
      settings: infoedit="Adder or subtractor-based accumulator.   Output type and binary point position match the input.<P><P>Hardware notes: When \"Reinitialize with input 'b' on reset\" is selected, the accumulator is forced to run at the system rate even if the input 'b' is running at a slower rate."  xl_area=[35 33 0 68 0 0 0]  block_version=10.1.2
  Constant : Constant  Value=0
  Convert : xbsIndex_r4/Convert  arith_type=Unsigned  n_bits=1  bin_pt=0  quantization=Truncate  overflow=Wrap  latency=0  dbl_ovrd=off  pipeline=off  block_type=convert
      settings: xl_area=[0 0 0 0 0 0 0]  block_version=10.1.2
  Convert1 : xbsIndex_r4/Convert  arith_type=Unsigned  n_bits=32  bin_pt=0  quantization=Truncate  overflow=Saturate  latency=0  dbl_ovrd=off  pipeline=off  block_type=convert
      settings: xl_area=[16 0 0 31 0 0 0]  block_version=10.1.2
  Convert2 : xbsIndex_r4/Convert  arith_type=Unsigned  n_bits=32  bin_pt=0  quantization=Truncate  overflow=Saturate  latency=0  dbl_ovrd=off  pipeline=off  block_type=convert
      settings: xl_area=[16 0 0 31 0 0 0]  block_version=10.1.2
  Counter : xbsIndex_r4/Counter  cnt_type=Free Running  cnt_to=Inf  operation=Up  start_count=0  cnt_by_val=1  arith_type=Unsigned  n_bits=1  bin_pt=0  load_pin=off  rst=off  en=off  explicit_period=on  period=1/8  dbl_ovrd=off  use_behavioral_HDL=off  use_rpm=off  block_type=counter
      settings: block_version=10.1.2
  Down Sample : xbsIndex_r4/Down Sample  sample_ratio=4  sample_phase="Last Value of Frame  (most efficient)"  en=off  latency=1  dbl_ovrd=off  block_type=dsamp
      settings: block_version=10.1.2
  Logical : xbsIndex_r4/Logical  logical_function=OR  inputs=2  en=off  latency=0  precision=Full  arith_type=Unsigned  n_bits=16  bin_pt=0  align_bp=on  dbl_ovrd=off  block_type=logical
      settings: xl_area=[1 0 0 1 0 0 0]  block_version=10.1.2
  Mux : xbsIndex_r4/Mux  inputs=2  en=off  latency=0  precision=Full  arith_type=Unsigned  n_bits=16  bin_pt=14  quantization=Truncate  overflow=Wrap  dbl_ovrd=off  block_type=mux
      settings: xl_area=[1 0 0 2 0 0 0]  block_version=10.1.2
  Negate : xbsIndex_r4/Negate  precision=Full  arith_type="Signed  (2's comp)"  n_bits=16  bin_pt=14  quantization=Truncate  overflow=Wrap  en=off  latency=0  dbl_ovrd=off  block_type=negate
      settings: xl_area=[1 0 0 2 0 0 0]  block_version=10.1.2
  OTRA : xbsIndex_r4/Gateway In  arith_type=Unsigned  n_bits=1  bin_pt=0  quantization="Round  (unbiased: +/- Inf)"  overflow=Saturate  period=1/8  dbl_ovrd=off  timing_constraint=None  locs_specified=off  LOCs={}  block_type=gatewayin
      settings: infoedit="Gateway in block.  Converts inputs of type Simulink integer, double and fixed point to  Xilinx fixed point type.<P><P>Hardware notes:  In hardware these blocks become top level input ports."  xl_area=[0 0 0 0 1 0 0]  block_version=10.1.2
  OTRB : xbsIndex_r4/Gateway In  arith_type=Unsigned  n_bits=1  bin_pt=0  quantization="Round  (unbiased: +/- Inf)"  overflow=Saturate  period=1/8  dbl_ovrd=off  timing_constraint=None  locs_specified=off  LOCs={}  block_type=gatewayin
      settings: infoedit="Gateway in block.  Converts inputs of type Simulink integer, double and fixed point to  Xilinx fixed point type.<P><P>Hardware notes:  In hardware these blocks become top level input ports."  xl_area=[0 0 0 0 1 0 0]  block_version=10.1.2
  RSSI : xbsIndex_r4/Gateway In  arith_type=Unsigned  n_bits=10  bin_pt=0  quantization="Round  (unbiased: +/- Inf)"  overflow=Saturate  period=1/8  dbl_ovrd=off  timing_constraint=None  locs_specified=off  LOCs={}  block_type=gatewayin
      settings: infoedit="Gateway in block.  Converts inputs of type Simulink integer, double and fixed point to  Xilinx fixed point type.<P><P>Hardware notes:  In hardware these blocks become top level input ports."  xl_area=[0 0 0 0 1 0 0]  block_version=10.1.2
  RSSI_CLK : xbsIndex_r4/Gateway Out  hdl_port=on  timing_constraint=None  locs_specified=off  LOCs={}  block_type=gatewayout
      settings: infoedit="Gateway out block.  Converts Xilinx fixed point inputs into ouputs of type Simulink integer, double, or fixed point.<P><P>Hardware notes:  In hardware these blocks become top level output ports or are discarded, depending on how they are configured."  block_version=10.1.2
  Register : xbsIndex_r4/Register  init=0  rst=off  en=off  dbl_ovrd=off  block_type=register
      settings: block_version=10.1.2
  Scope : Scope
  Up Sample : xbsIndex_r4/Up Sample  sample_ratio=4  copy_samples=on  dbl_ovrd=off  block_type=usamp
      settings: infoedit="Up samples input data.  Inserted values  can be zeros or copies of the most recent input sample.<P><P>Hardware notes: No hardware is needed if inserted values are copies of the input sample; otherwise, a mux and single bit flip-flop are used."  block_version=10.1.2
  tag scope: OTR=global, RSSI=global
  wires:
  OTRA/1 -> Logical/1
  OTRB/1 -> Logical/2
  Logical/1 -> Convert/1
  Convert/1 -> Mux/1
  Mux/1 -> Accumulator/1
  [BENEFIT] -> Mux/2
  [COST] -> Negate/1
  Negate/1 -> Mux/3
  Constant/1 -> OTRA/1, OTRB/1
  Accumulator/1 -> Convert1/1
  RSSI/1 -> Down Sample/1
  Down Sample/1 -> Register/1
  Register/1 -> Convert2/1
  Convert1/1 -> [OTR]
  Convert2/1 -> Up Sample/1
  Up Sample/1 -> [RSSI]
  Counter/1 -> RSSI_CLK/1
  RSSI_CLK/1 -> Scope/1
